simulink subsystem "energy_distribution"  (R2024a)
settings: Solver=VariableStepAuto  StartTime=0.0  StopTime=10.0  RelTol=1e-3
undefined symbols (not defined in the file): I_batt_max, I_batt_min, I_gen_max, I_gen_min, Ki, NLF_alpha1, SoC_min, tau_gen, V_nom
libraries: slpidlib x1
settings Model: Creator=User  LastModifiedBy=Henrique Mesquita

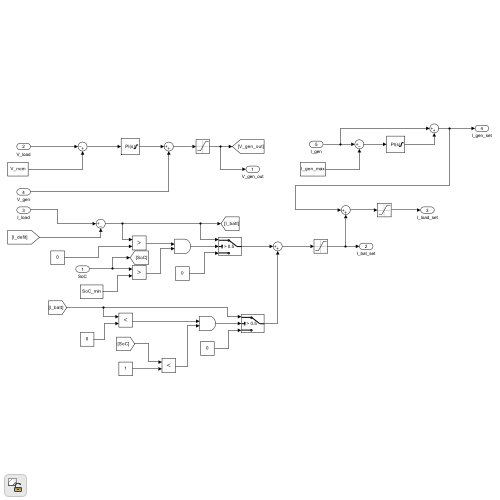
[thumbnail: Simulink's stored preview of the top-level diagram]
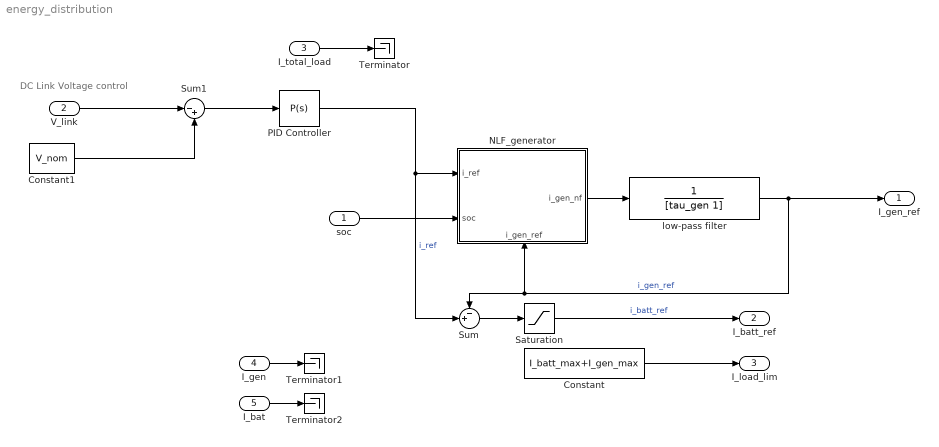
== system energy_distribution ==
  note: DC Link Voltage control
  soc : Inport
  V_link : Inport  Port=2
  I_total_load : Inport  Port=3
  I_gen : Inport  Port=4
  I_bat : Inport  Port=5
  Constant : Constant  Value=I_batt_max+I_gen_max
  Constant1 : Constant  Value=V_nom
  NLF_generator : Subsystem
      settings: PortSchema="{\"entries\":[{\"content\":{\"sides\":[{\"content\":{\"connectorIds\":[\"In1\",\"In2\"]},\"type\":\"ConnectorPlacement.EquallySpacedRectSide\",\"uuid\":\"174a34ca-0ae7-4c78-a365-6d5b22c651bf\"},{\"content\":{\"connectorIds\":[\"Out1\"],\"side\":\"RIGHT\"},\"type\":\"ConnectorPlacement.EquallySpacedRectSide\",\"uuid\":\"bf3ae82c-8e63-482a-a9f1-1bb59725503e\"},{\"content\":{\"side\":\"TOP\"},\"type\":\"ConnectorPlacement.EquallySpacedRectSide\",\"uuid\":\"9e312b37-d84c-41db-afb0-7e0273bdd53c\"},{\"content\":{\"connectorIds\":[\"In3\"],\"side\":\"BOTTOM\"},\"type\":\"ConnectorPlacement.EquallySpacedRectSide\",\"uuid\":\"40d0a9ba-eb32-4d3b-a0b8-1bb7bbf43618\"}]},\"type\":\"ConnectorPlacement.EquallySpacedConnector\",\"uuid\":\"477f26ea-72e0-47af-ab47-e4b9bc1e1d78\"}],\"packageUris\":[\"http://schema.mathworks.com/mf0/Connector/R2020b\"],\"version\":\"1.0\"}"
  PID Controller : slpidlib/PID Controller  Controller=P  Form=Parallel  TimeDomain=Continuous-time  UseExternalTs=off  SampleTime=-1  IntegratorMethod=Forward Euler  FilterMethod=Forward Euler  ControllerParametersSource=internal  P=20  I=Ki  UseKiTs=off  D=0  UseExternalDerivativeSource=off  N=100  UseFilter=on  TunerSelectOption=Transfer Function Based (PID Tuner App)  InitialConditionSource=internal  InitialConditionForIntegrator=0  InitialConditionForFilter=0  DifferentiatorICPrevScaledInput=0  ExternalReset=none  TrackingMode=off  Kt=1  LimitOutput=on  SatLimitsSource=internal  UpperSaturationLimit=inf  LowerSaturationLimit=-inf  LinearizeAsGain=on  AntiWindupMode=back-calculation  Kb=2  LimitIntegrator=off  UpperIntegratorSaturationLimit=inf  LowerIntegratorSaturationLimit=-inf  POutMin=[]  POutMax=[]  IOutMin=[]  IOutMax=[]  DOutMin=[]  DOutMax=[]  NOutMin=[]  NOutMax=[]  SumOutMin=[]  SumOutMax=[]  SaturationOutMin=[]  SaturationOutMax=[]  PParamMin=[]  PParamMax=[]  IParamMin=[]  IParamMax=[]  DParamMin=[]  DParamMax=[]  NParamMin=[]  NParamMax=[]  KbParamMin=[]  KbParamMax=[]  KtParamMin=[]  KtParamMax=[]  KbOutMin=[]  KbOutMax=[]  KtOutMin=[]  KtOutMax=[]  IntegratorOutMin=[]  IntegratorOutMax=[]  FilterOutMin=[]  FilterOutMax=[]  SumI1OutMin=[]  SumI1OutMax=[]  SumI2OutMin=[]  SumI2OutMax=[]  SumI3OutMin=[]  SumI3OutMax=[]  SumI4OutMin=[]  SumI4OutMax=[]  SumDOutMin=[]  SumDOutMax=[]  DifferentiatorOutMin=[]  DifferentiatorOutMax=[]  FilterDiffOutCoefMin=[]  FilterDiffOutCoefMax=[]  ReciprocalOutMin=[]  ReciprocalOutMax=[]  SumDenOutMin=[]  SumDenOutMax=[]  SumNumOutMin=[]  SumNumOutMax=[]  DivideOutMin=[]  DivideOutMax=[]  UdiffTsProdOutMin=[]  UdiffTsProdOutMax=[]  NTsProdOutMin=[]  NTsProdOutMax=[]  UintegralTsProdOutMin=[]  UintegralTsProdOutMax=[]  UngainTsProdOutMin=[]  UngainTsProdOutMax=[]  ClampingZeroOutDataTypeStr=Inherit: Inherit via back propagation  ClampingZeroOutMin=[]  ClampingZeroOutMax=[]  FilterDenConstantOutDataTypeStr=Inherit: Inherit via back propagation  FilterDenConstantOutMin=[]  FilterDenConstantOutMax=[]  PCopyOutDataTypeStr=Inherit: Inherit via back propagation  PCopyOutMin=[]  PCopyOutMax=[]  NCopyOutDataTypeStr=Inherit: Inherit via back propagation  NCopyOutMin=[]  NCopyOutMax=[]  IntegratorContinuousStateAttributes=''  IntegratorStateMustResolveToSignalObject=off  IntegratorRTWStateStorageClass=Auto  FilterContinuousStateAttributes=''  FilterStateMustResolveToSignalObject=off  FilterRTWStateStorageClass=Auto  ParallelPVariant=InternalParameters  IdealPVariant=Disabled  IVariant=Disabled  DVariant=Disabled  IntegratorVariant=Disabled  SatVariant=Enabled  AWVariant=Disabled  PCopyVariant=Disabled  TRVariant=Disabled  FdbkBlocksVariant=Forward  IdealPFdbkVariant=Disabled  SatFdbkVariant=Disabled  DerivativeFilterVariant=Disabled  NVariant=Disabled  NCopyVariant=Disabled_SignalSpec  FilterICVariant=Disabled  IntegratorICVariant=Disabled  ExternalResetVariant=Disabled  TRSumVariant=Passthrough  SumFdbkVariant=Disabled  SumVariant=Passthrough_P  TsampFilterVariant=InternalTs  TsampNgainVariant=Passthrough  TsampIntegralVariant=Disabled_SignalSpec  ExternalSaturationOutDataTypeStr=Inherit: Same as second input  DerivativeSourceVariant=Disabled
  Saturation : Saturate  UpperLimit=I_batt_max  LowerLimit=I_batt_min
  Sum : Sum  Inputs=-+|
  Sum1 : Sum  Inputs=|-+
  Terminator : Terminator
  Terminator1 : Terminator
  Terminator2 : Terminator
  low-pass filter : TransferFcn  Denominator=[tau_gen 1]
  I_gen_ref : Outport
  I_batt_ref : Outport  Port=2
  I_load_lim : Outport  Port=3
  wires:
  Constant/1 -> I_load_lim/1
  low-pass filter/1 -> NLF_generator/3(i_gen_ref), Sum/1, I_gen_ref/1  "i_gen_ref"
  Saturation/1 -> I_batt_ref/1  "i_batt_ref"
  soc/1 -> NLF_generator/2(soc)
  NLF_generator/1(i_gen_nf) -> low-pass filter/1
  PID Controller/1 -> NLF_generator/1(i_ref), Sum/2  "i_ref"
  Sum/1 -> Saturation/1
  Sum1/1 -> PID Controller/1
  Constant1/1 -> Sum1/2
  V_link/1 -> Sum1/1
  I_total_load/1 -> Terminator/1
  I_gen/1 -> Terminator1/1
  I_bat/1 -> Terminator2/1

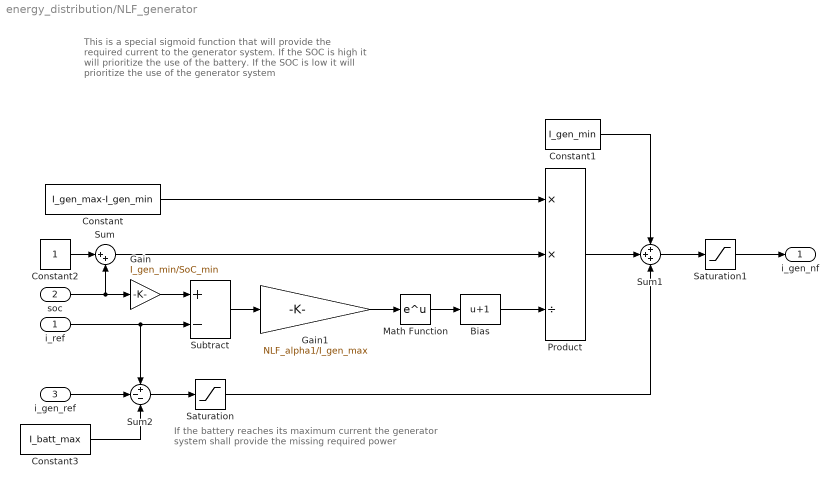
== system energy_distribution/NLF_generator ==
  note: This is a special sigmoid function that will provide the required current to the generator system. If the SOC is high it will prioritize the use of the battery. If the SOC is low it will prioritize the use of the generator system
  note: If the battery reaches its maximum current the generator system shall provide the missing required power
  i_ref : Inport
  soc : Inport  Port=2
  i_gen_ref : Inport  Port=3
  Bias : Bias  Bias=1  SaturateOnIntegerOverflow=off
  Constant : Constant  Value=I_gen_max-I_gen_min
  Constant1 : Constant  Value=I_gen_min
  Constant2 : Constant
  Constant3 : Constant  Value=I_batt_max
  Gain : Gain  Gain=I_gen_min/SoC_min
  Gain1 : Gain  Gain=NLF_alpha1/I_gen_max
  Math Function : Math
  Product : Product  Inputs=**/
  Saturation : Saturate  UpperLimit=Inf  LowerLimit=0
  Saturation1 : Saturate  UpperLimit=I_gen_max  LowerLimit=I_gen_min
  Subtract : Sum  Inputs=+-
  Sum : Sum  Inputs=|++
  Sum1 : Sum  Inputs=+++
  Sum2 : Sum  Inputs=+--
  i_gen_nf : Outport
  wires:
  Saturation1/1 -> i_gen_nf/1
  Saturation/1 -> Sum1/3
  Sum2/1 -> Saturation/1
  Constant3/1 -> Sum2/3
  i_gen_ref/1 -> Sum2/2
  Constant1/1 -> Sum1/1
  Sum1/1 -> Saturation1/1
  Product/1 -> Sum1/2
  Constant/1 -> Product/1
  Sum/1 -> Product/2
  Bias/1 -> Product/3
  Gain1/1 -> Math Function/1
  Subtract/1 -> Gain1/1
  i_ref/1 -> Subtract/2, Sum2/1
  Gain/1 -> Subtract/1
  soc/1 -> Sum/2, Gain/1
  Constant2/1 -> Sum/1
  Math Function/1 -> Bias/1
